simulink model "CalcSubSys"  (R2020a)
settings: Solver=FixedStepDiscrete  StartTime=0.0  StopTime=10.0  RelTol=1e-3
settings Model: Creator=yomna  LastModifiedBy=yomna
settings OptimizationCC: DefaultParameterBehavior=Inlined  EnhancedBackFolding=on  PassReuseOutputArgsAs=Individual arguments  ZeroExternalMemoryAtStartup=off  ZeroInternalMemoryAtStartup=off  OptimizeBlockOrder=speed  DifferentSizesBufferReuse=on  OptimizationCustomize=off  EfficientTunableParamExpr=on
settings DebuggingCC: UnderspecifiedInitializationDetection=Classic  MergeDetectMultiDrivingBlocksExec=none  ParameterTunabilityLossMsg=error
settings ModelReferenceCC: PropagateSignalLabelsOutOfModel=off
settings SFSimCC: MATLABDynamicMemAlloc=off
settings RTWCC: SystemTargetFile=ert.tlc  GenCodeOnly=on  TemplateMakefile=ert_default_tmf  GenerateReport=on  IncludeHyperlinkInReport=on  LaunchReport=on  GenerateTraceInfo=on  GenerateTraceReport=on  GenerateTraceReportSl=on  GenerateTraceReportSf=on  GenerateTraceReportEml=on
settings CodeAppCC: ForceParamTrailComments=on  IgnoreCustomStorageClasses=off  OperatorAnnotations=on  SimulinkDataObjDesc=on  SFDataObjDesc=on  InsertBlockDesc=on
settings ERTTargetCC: TargetLangStandard=C99 (ISO)  GenerateSampleERTMain=on  InlinedParameterPlacement=NonHierarchical  ERTCustomFileTemplate=example_file_process.tlc

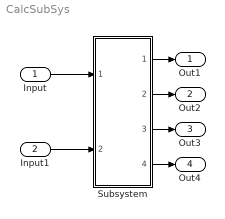
== system CalcSubSys ==
  Input : Inport
  Input1 : Inport  Port=2
  Subsystem : Subsystem
  Out1 : Outport
  Out2 : Outport  Port=2
  Out3 : Outport  Port=3
  Out4 : Outport  Port=4
  wires:
  Input1/1 -> Subsystem/2(Input1)
  Subsystem/3(Out3) -> Out3/1
  Subsystem/1(Out1) -> Out1/1
  Subsystem/4(Out4) -> Out4/1
  Input/1 -> Subsystem/1(Input)
  Subsystem/2(Out2) -> Out2/1

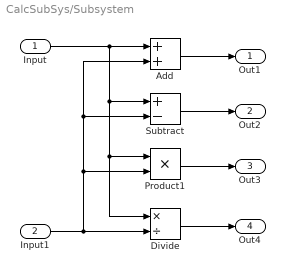
== system CalcSubSys/Subsystem ==
  Input : Inport  OutDataTypeStr=int32
  Input1 : Inport  Port=2  OutDataTypeStr=int32
  Add : Sum
  Divide : Product  Inputs=*/
  Product1 : Product
  Subtract : Sum  Inputs=+-
  Out1 : Outport
  Out2 : Outport  Port=2
  Out3 : Outport  Port=3
  Out4 : Outport  Port=4
  wires:
  Product1/1 -> Out3/1
  Input1/1 -> Add/2, Subtract/2, Product1/2, Divide/2
  Input/1 -> Divide/1, Product1/1, Subtract/1, Add/1
  Divide/1 -> Out4/1
  Subtract/1 -> Out2/1
  Add/1 -> Out1/1
